simulink model "fahrenheitConverter_NicholasSeecharan"  (R2025b)
settings: Solver=VariableStepAuto  StartTime=0.0  StopTime=10.0  RelTol=1e-3

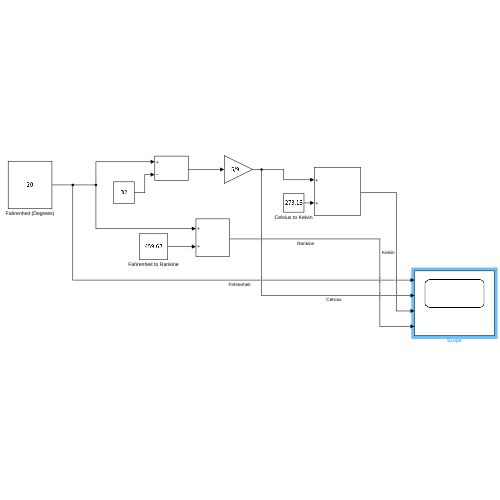
[thumbnail: Simulink's stored preview of the top-level diagram]
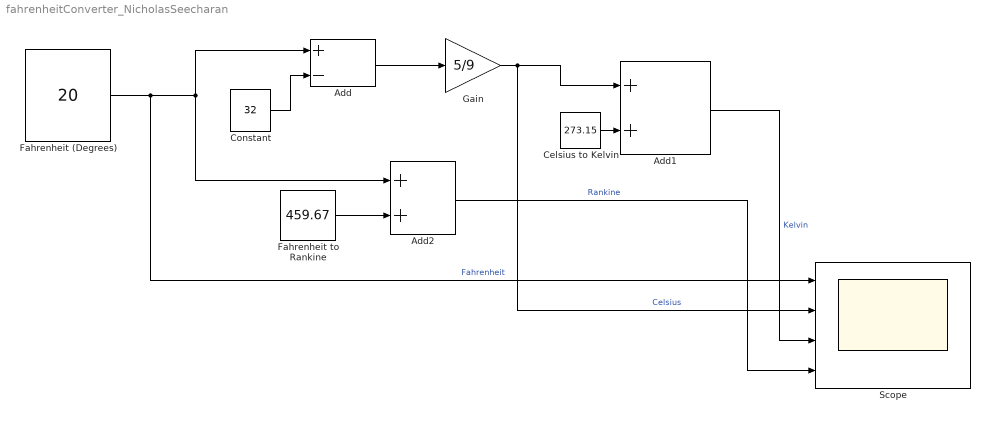
== system fahrenheitConverter_NicholasSeecharan ==
  Add : Sum  Inputs=+-
  Add1 : Sum
  Add2 : Sum
  Celsius to Kelvin : Constant  Value=273.15
  Constant : Constant  Value=32
  Fahrenheit (Degrees) : Constant  Value=20
  Fahrenheit to Rankine : Constant  Value=459.67
  Gain : Gain  Gain=5/9
  Scope : Scope  NumInputPorts=4
      settings: SampleTime=10  ActiveDisplayYMaximum=500
  wires:
  Fahrenheit (Degrees)/1 -> Scope/1, Add2/1, Add/1  "Fahrenheit"
  Constant/1 -> Add/2
  Add/1 -> Gain/1
  Gain/1 -> Scope/2, Add1/1  "Celsius"
  Celsius to Kelvin/1 -> Add1/2
  Fahrenheit to Rankine/1 -> Add2/2
  Add1/1 -> Scope/3  "Kelvin"
  Add2/1 -> Scope/4  "Rankine"
